simulink model "NCGPC_BoucleOuverte"  (R2016b)
settings: Solver=ode5  StartTime=0.0  StopTime=30  FixedStep=0.005  RelTol=1e-2
libraries: simulink x1
settings Model: Creator=amar  LastModifiedBy=fnadi

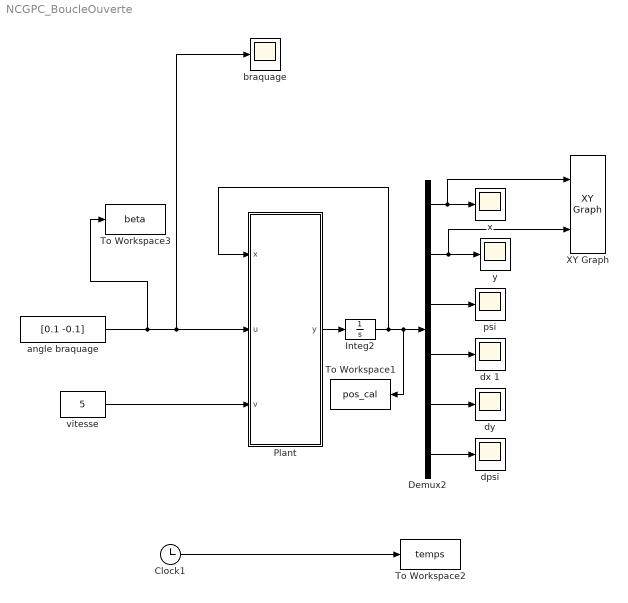
== system NCGPC_BoucleOuverte ==
  Clock1 : Clock
  Demux2 : Demux  Outputs=6
  Integ2 : Integrator  InitialCondition="[0 0 -pi/3*0 5 0  0]"
  Plant : MATLAB Function  TreatAsAtomicUnit=on
  To Workspace1 : ToWorkspace  VariableName=pos_cal  SampleTime=-1
  To Workspace2 : ToWorkspace  VariableName=temps  SampleTime=-1
  To Workspace3 : ToWorkspace  VariableName=beta  SampleTime=-1
  XY Graph : simulink/Sinks/XY Graph  xmin=-50  xmax=50  ymin=-50  ymax=50  st=-1
  angle braquage : Constant  Value=[0.1 -0.1]
  braquage : Scope
  dpsi : Scope
  dx 1 : Scope
  dy : Scope
  psi : Scope
  vitesse : Constant  Value=5
  "x " : Scope
  "y " : Scope
  wires:
  Plant/1(y) -> Integ2/1
  Demux2/5 -> dy/1
  Demux2/6 -> dpsi/1
  Demux2/4 -> dx 1/1
  Demux2/3 -> psi/1
  Demux2/2 -> XY Graph/2, "y "/1
  Demux2/1 -> XY Graph/1, "x "/1
  Integ2/1 -> Plant/1(x), To Workspace1/1, Demux2/1
  vitesse/1 -> Plant/3(v)
  angle braquage/1 -> To Workspace3/1, Plant/2(u), braquage/1
  Clock1/1 -> To Workspace2/1

== matlab function NCGPC_BoucleOuverte/Plant ==
  data: x input; u input; v input; y output
function y = plant(x,u,v)

%global param

%rigidité de dérive
Cf=10000;
Cr=10000;

%position du cdg
a=1.2;
b=1.2;

%masse et momet d'inertie
masse=700;
moment=400*(1.2^2+0.7^2)/12;

%vitesse
vit=v;

%%
beta_f=u(1);
beta_r=u(2);

Xpos=x(1);
Ypos=x(2);
psi=x(3);

dXpos=x(4);
dYpos=x(5);
dpsi=x(6);

%% matrice A et B
a11=-2*(Cf+Cr)/(masse*vit);
a12=-2*(a*Cf-b*Cr)/(masse*vit)+vit;
a21=-2*(a*Cf-b*Cr)/(vit*moment);
a22=-2*(a^2*Cf+b^2*Cr)/(vit*moment);

b11=2*Cf/masse; b12=2*Cr/masse;
b21=2*a*Cf/moment; b22=-2*b*Cr/moment;

%%

R=[cos(psi) -sin(psi); sin(psi) cos(psi)];

V = R'*[dXpos; dYpos];
Vx=V(1);
Vy=V(2);

%%

dVx =0 ;
dVy = a11*Vy + a12*dpsi + b11*beta_f + b12*beta_r;
ddpsi = a21*Vy + a22*dpsi + b21*beta_f + b22*beta_r;

%%

acc = R*[dVx; dVy] + dpsi*[-Vx*sin(psi)-Vy*cos(psi); Vx*cos(psi)-Vy*sin(psi)] ;

ddXpos=acc(1); 
ddYpos=acc(2);

y = [x(4) x(5) x(6) ddXpos ddYpos ddpsi] ;
